simulink model "model"  (R2013a)
settings: Solver=ode4  StartTime=0.0  StopTime=time  FixedStep=0.001  MaxStep=2  MinStep=0.01  RelTol=1e-3
values from neighbouring files (symbols this model uses):
  ep = 0.005    [main.m]
  y_zad = 1    [main.m]
libraries: cstblocks x1
settings Model: Creator=Michał Strada  LastModifiedBy=Michał Strada

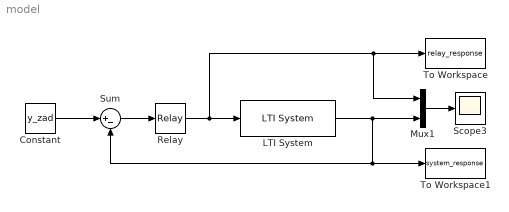
== system model ==
  Constant : Constant  Value=y_zad
  LTI System : cstblocks/LTI System  sys=G  IC=[]
  Mux1 : Mux  Inputs=2
  Relay : Relay  OnSwitchValue=ep  OffSwitchValue=-ep  OffOutputValue=-1
  Scope3 : Scope
      settings: MaxDataPoints=500000
  Sum : Sum  Inputs=|+-
  To Workspace : ToWorkspace  VariableName=relay_response  SampleTime=-1  SaveFormat=Timeseries
  To Workspace1 : ToWorkspace  VariableName=system_response  SampleTime=-1  SaveFormat=Timeseries
  wires:
  Constant/1 -> Sum/1
  Sum/1 -> Relay/1
  LTI System/1 -> Mux1/2, Sum/2, To Workspace1/1
  Mux1/1 -> Scope3/1
  Relay/1 -> To Workspace/1, Mux1/1, LTI System/1
